simulink model "zad_1"  (R2023b)
settings: Solver=VariableStepAuto  StartTime=0.0  StopTime=10.0  RelTol=1e-3
settings Model: Creator=matiz  LastModifiedBy=matiz

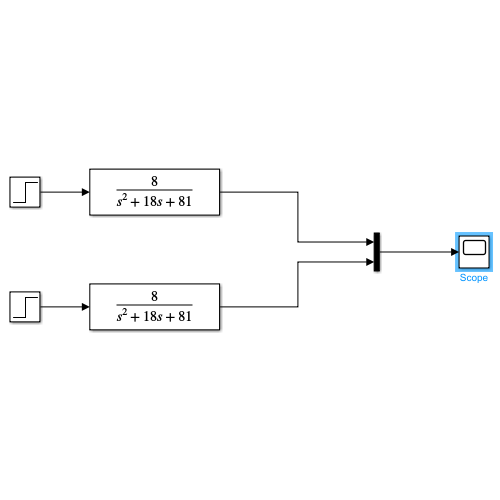
[thumbnail: Simulink's stored preview of the top-level diagram]
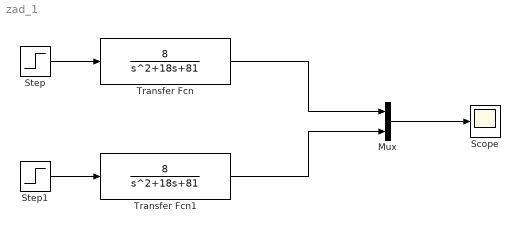
== system zad_1 ==
  Mux : Mux  Inputs=2
  Scope : Scope
  Step : Step  SampleTime=0
  Step1 : Step  After=5  SampleTime=0
  Transfer Fcn : TransferFcn  Numerator=[8]  Denominator=[1 18 81]
  Transfer Fcn1 : TransferFcn  Numerator=[8]  Denominator=[1 18 81]
  wires:
  Step/1 -> Transfer Fcn/1
  Step1/1 -> Transfer Fcn1/1
  Transfer Fcn/1 -> Mux/1
  Transfer Fcn1/1 -> Mux/2
  Mux/1 -> Scope/1
